simulink model "fcn_test"  (Simulink 8.4)
settings: Solver=VariableStepDiscrete  StartTime=0.0  StopTime=1  MaxStep=1  RelTol=1e-3
settings Model: Creator=arnaud  LastModifiedBy=arnaud
settings DataIOCC: SaveFormat=Structure  SignalLoggingSaveFormat=Dataset
settings OptimizationCC: ExpressionDepthLimit=128
settings DebuggingCC: UnderspecifiedInitializationDetection=Simplified  MergeDetectMultiDrivingBlocksExec=error  FcnCallInpInsideContextMsg=EnableAllAsError  StateNameClashWarn=none
settings GRTTargetCC: CombineOutputUpdateFcns=on  GRTInterface=off

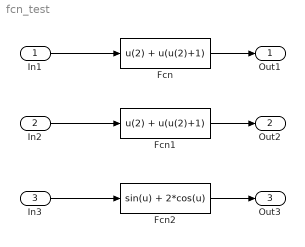
== system fcn_test ==
  In1 : Inport  PortDimensions=[1 3]
  In2 : Inport  Port=2  PortDimensions=2
  In3 : Inport  Port=3  PortDimensions=2
  Fcn : Fcn  Expr=u(2) + u(u(2)+1)
  Fcn1 : Fcn  Expr=u(2) + u(u(2)+1)
  Fcn2 : Fcn  Expr=sin(u) + 2*cos(u)
  Out1 : Outport
  Out2 : Outport  Port=2
  Out3 : Outport  Port=3
  wires:
  Fcn/1 -> Out1/1
  In1/1 -> Fcn/1
  Fcn1/1 -> Out2/1
  In2/1 -> Fcn1/1
  Fcn2/1 -> Out3/1
  In3/1 -> Fcn2/1
